simulink model "stage12"  (Simulink 7.7)
settings: Solver=ode45  StartTime=0.0  StopTime=2  RelTol=1e-3
undefined symbols (not defined in the file): Acid, idx_data, iv_data, Lead
libraries: powerlib x23, simulink x4, fl_lib x4, nesl_utility x3, powerlib_extras x2, electricdrivelib x2, elec_lib x2
settings Model: Creator=Vikas  LastModifiedBy=HASANTH

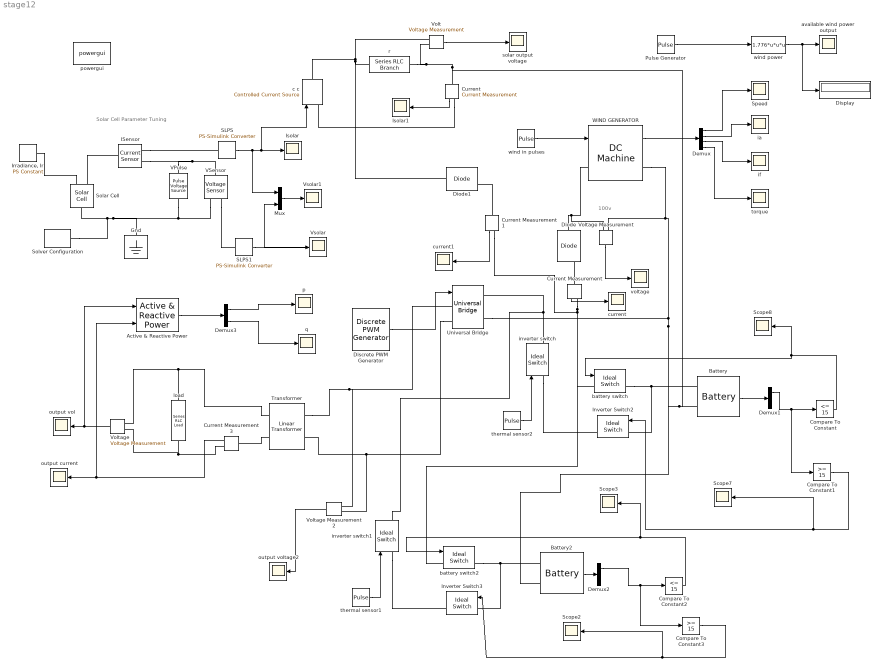
== system stage12 ==
  note: 100v
  note: Solar Cell Parameter Tuning
  Active & Reactive Power : powerlib_extras/Measurements/Active & Reactive Power  SystemSampleTime=-1  f1=50
  Battery : electricdrivelib/Extra Sources/Battery  SystemSampleTime=-1  BatType=Lead-Acid  ShowDetailedParameters=off  NomV=15  NomQ=60  SOC=0  PresetModel=on  MaxQ=62.5  FullV=16.3322  Dis_rate=12  R=0.0025  Normal_OP=18.6167  expZone="[15.2714          0.2]"  Dis_Char=off  current=[6.5 13 32.5]  Units=Time  Batt_Tr=5
  Battery2 : electricdrivelib/Extra Sources/Battery  SystemSampleTime=-1  BatType=Lead-Acid  ShowDetailedParameters=off  NomV=15  NomQ=60  SOC=100  PresetModel=on  MaxQ=62.5  FullV=16.3322  Dis_rate=12  R=0.0025  Normal_OP=18.6167  expZone="[15.2714          0.2]"  Dis_Char=off  current=[6.5 13 32.5]  Units=Time  Batt_Tr=5
  Compare To Constant : simulink/Logic and Bit Operations/Compare To Constant  SystemSampleTime=-1  relop=<=  const=15  LogicOutDataTypeMode=uint8
  Compare To Constant1 : simulink/Logic and Bit Operations/Compare To Constant  SystemSampleTime=-1  relop=>=  const=15  LogicOutDataTypeMode=uint8
  Compare To Constant2 : simulink/Logic and Bit Operations/Compare To Constant  SystemSampleTime=-1  relop=<=  const=15  LogicOutDataTypeMode=uint8
  Compare To Constant3 : simulink/Logic and Bit Operations/Compare To Constant  SystemSampleTime=-1  relop=>=  const=15  LogicOutDataTypeMode=uint8
  Current : powerlib/Measurements/Current Measurement  SystemSampleTime=-1  PhasorSimulation=off  OutputType=Complex  PSBequivalent=0
  Current Measurement : powerlib/Measurements/Current Measurement  SystemSampleTime=-1  PhasorSimulation=off  OutputType=Complex  PSBequivalent=0
  Current Measurement1 : powerlib/Measurements/Current Measurement  SystemSampleTime=-1  PhasorSimulation=off  OutputType=Complex  PSBequivalent=0
  Current Measurement3 : powerlib/Measurements/Current Measurement  SystemSampleTime=-1  PhasorSimulation=off  OutputType=Complex  PSBequivalent=0
  Demux : Demux
  Demux1 : Demux  Outputs=3
  Demux2 : Demux  Outputs=3
  Demux3 : Demux  Outputs=2
  Diode : powerlib/Power Electronics/Diode  SystemSampleTime=-1  Ron=0.001  Lon=0  Vf=0.8  IC=0  UseSnubber=off  Rs=500  Cs=250e-9  Measurements=on
  Diode1 : powerlib/Power Electronics/Diode  SystemSampleTime=-1  Ron=0.001  Lon=0  Vf=0.8  IC=0  UseSnubber=off  Rs=500  Cs=250e-9  Measurements=on
  Discrete PWM Generator : powerlib_extras/Discrete  Control Blocks/Discrete PWM Generator  SystemSampleTime=-1  GeneratorMode="2-arm  bridge (4 pulses)"  Fc=1080  Ts=5e-6  Internal=on  mIndex=0.4  Freq=50  Phase=0
  Display : Display
  Gnd : fl_lib/Electrical/Electrical Elements/Electrical Reference  SystemSampleTime=-1  i_Log=off  LocalVarNames=|i  LocalVarDescs=|i  LocalVarLogging=[]
  ISensor : fl_lib/Electrical/Electrical Sensors/Current Sensor  SystemSampleTime=-1  i1_Log=off  v1_Log=off  LocalVarNames=|i1|v1  LocalVarDescs=|i1|v1  LocalVarLogging=[0 0]
  Inverter Switch2 : powerlib/Power Electronics/Ideal Switch  SystemSampleTime=-1  Ron=0.001  Lon=0  IC=0  Rs=1e5  Cs=inf  Measurements=on
  Inverter Switch3 : powerlib/Power Electronics/Ideal Switch  SystemSampleTime=-1  Ron=0.001  Lon=0  IC=0  Rs=1e5  Cs=inf  Measurements=on
  "Irradiance, Ir" : fl_lib/Physical Signals/Sources/PS Constant  SystemSampleTime=-1  constant=1000  LocalVarLogging=[]
  Isolar : Scope
      settings: TimeRange=1  YMin=2.23577  YMax=2.23577  SaveName=Io
  Isolar1 : Scope
      settings: TimeRange=1  YMin=2.23577  YMax=2.23577  SaveName=Io1
  Mux : Mux  Inputs=2
  Pulse Generator : DiscretePulseGenerator  PulseType=Time based  Amplitude=3.84  Period=10  PulseWidth=50
  SLPS : nesl_utility/PS-Simulink Converter  SystemSampleTime=-1  PhysicalDomain=network_engine_domain  LeftPortType=input  RightPortType=output  SubClassName=ps_output  Unit=A  AffineConversion=off
  SLPS1 : nesl_utility/PS-Simulink Converter  SystemSampleTime=-1  PhysicalDomain=network_engine_domain  LeftPortType=input  RightPortType=output  SubClassName=ps_output  Unit=V  AffineConversion=off
  Scope{2..3,7..8} (4 alike) : Scope
      Scope2 settings: TimeRange=0.1  YMin=0.95  YMax=1.05  SaveName=ScopeData5
      Scope3 settings: TimeRange=0.02  YMin=0.95  YMax=1.05  SaveName=ScopeData10
      Scope7 settings: TimeRange=0.1  YMin=0.95  YMax=1.05  SaveName=ScopeData7
      Scope8 settings: TimeRange=0.02  YMin=0.95  YMax=1.05  SaveName=ScopeData9
  Solar Cell : elec_lib/Sources/Solar Cell  SystemSampleTime=-1  prm=1  Isc=7.34 A  Voc=0.6 V  Is=1e-06 A  Is2=0 A  Iph=7.34 A  Ir0=1000 W/m^2  ec=1.5  N2=2  Rs=0 Ohm  Rp=Inf Ohm  TIPH1=0 1/K  EG=1.11 eV  TXIS1=3  TXIS2=3  TRS1=0  TRP1=0  TFIXED=iv_data(idx_data).temperature C  Tmeas=25 C  LocalVarLogging=[]
  Solver Configuration : nesl_utility/Solver Configuration  SystemSampleTime=-1  PhysicalDomain=network_engine_domain  LeftPortType=input  RightPortType=generic  SubClassName=solver  Accelerate=off  Profile=off  ResidualTolerance=1e-9  MaxNonlinIter=3  MaxModeIter=2  DoFixedCost=off  UseLocalSampling=off  DoDC=off  LinearAlgebra=Sparse  LocalSolverSampleTime=.001  LocalSolverChoice=NE_BACKWARD_EULER_ADVANCER  UseLocalSolver=off
  Speed : Scope
      settings: YMin=5.3  YMax=5.3
  Transformer : powerlib/Elements/Linear Transformer  PhysicalDomain=powersysdomain  SubClassName=unknown  LeftPortType=p1  RightPortType=p1  LConnTagsString=a|b  RConnTagsString=A|B  UNITS=pu  NominalPower=[ 875 50 ]  winding1=[12 0.002 0]  winding2=[240 0.002 0.0]  ThreeWindings=off  winding3=[3.15e+005 0.002 0.08]  RmLm=[500 500]  Measurements=None  DataType=off
  Universal Bridge : powerlib/Power Electronics/Universal Bridge  SystemSampleTime=-1  Arms=2  SnubberResistance=1e5  SnubberCapacitance=inf  Device=MOSFET / Diodes  Ron=1e-3  Lon=0  ForwardVoltages="[  0  0  ]"  ForwardVoltage=0  GTOparameters=[ 10e-6 , 20e-6 ]  IGBTparameters=[ 1e-6 , 2e-6 ]  Measurements=None  Measurements_2=None  converterType=Rectifier
  VPulse : elec_lib/Additional Components/SPICE-Compatible Components/Sources/Pulse Voltage Source  SystemSampleTime=-1  V1=0 V  V2=iv_data(idx_data).v(end) V  TD=0 s  TR=1 s  TF=0 s  PW=Inf s  PER=Inf s  voltage_Log=off  LocalVarNames=|voltage  LocalVarDescs=|Voltage (V)  LocalVarLogging=0
  VSensor : fl_lib/Electrical/Electrical Sensors/Voltage Sensor  SystemSampleTime=-1  i1_Log=off  v1_Log=off  LocalVarNames=|i1|v1  LocalVarDescs=|i1|v1  LocalVarLogging=[0 0]
  Volt : powerlib/Measurements/Voltage Measurement  SystemSampleTime=-1  PhasorSimulation=off  OutputType=Complex  PSBequivalent=0
  Voltage : powerlib/Measurements/Voltage Measurement  SystemSampleTime=-1  PhasorSimulation=off  OutputType=Complex  PSBequivalent=0
  Voltage Measurement : powerlib/Measurements/Voltage Measurement  SystemSampleTime=-1  PhasorSimulation=off  OutputType=Complex  PSBequivalent=0
  Voltage Measurement2 : powerlib/Measurements/Voltage Measurement  SystemSampleTime=-1  PhasorSimulation=off  OutputType=Complex  PSBequivalent=0
  Vsolar : Scope
      settings: TimeRange=1  YMin=0  YMax=0.8  SaveName=Vo
  Vsolar1 : Scope
      settings: TimeRange=1  YMin=0.5  YMax=2.3  SaveName=Vo1
  WIND GENERATOR : powerlib/Machines/DC Machine  SystemSampleTime=-1  PresetModel=No  MechanicalLoad=Speed w  FieldType=Permanent magnet  ShowDetailedParameters=on  RLa="[ 2  0.012]"  RLf="[ 240  120]"  Laf=1.8  MachineConstant=Back-emf constant (V/rpm)  Ke=3  Kt=3.18  J=1  Bm=0  Tf=0  w0=1  Ifinit=1  TsPowergui=0  TsBlock=-1
      settings: AttributesFormatString=\n
  available wind power output : Scope
      settings: TimeRange=0.1  YMin=265.673  YMax=293.639  SaveName=ScopeData13
  battery switch : powerlib/Power Electronics/Ideal Switch  SystemSampleTime=-1  Ron=0.001  Lon=0  IC=0  Rs=1e5  Cs=inf  Measurements=on
  battery switch2 : powerlib/Power Electronics/Ideal Switch  SystemSampleTime=-1  Ron=0.001  Lon=0  IC=0  Rs=1e5  Cs=inf  Measurements=on
  c c : powerlib/Electrical Sources/Controlled Current Source  SystemSampleTime=-1  Initialize=on  Source_Type=DC  Amplitude=1  Phase=0  Frequency=0  Measurements=None
  current : Scope
      settings: TimeRange=0.04  YMin=7.52429  YMax=7.52443  SaveName=ScopeData6
  current1 : Scope
      settings: TimeRange=0.04  YMin=7.21301  YMax=7.21303  SaveName=ScopeData11
  ia : Scope
      settings: YMin=-7.52695  YMax=-7.5266
  if : Scope
      settings: SaveName=ScopeData2
  inverter switch : powerlib/Power Electronics/Ideal Switch  SystemSampleTime=-1  Ron=0.001  Lon=0  IC=0  Rs=1e5  Cs=inf  Measurements=on
  inverter switch1 : powerlib/Power Electronics/Ideal Switch  SystemSampleTime=-1  Ron=0.001  Lon=0  IC=0  Rs=1e5  Cs=inf  Measurements=on
  load : powerlib/Elements/Series RLC Load  PhysicalDomain=powersysdomain  SubClassName=unknown  LeftPortType=p1  RightPortType=p1  LConnTagsString=a  RConnTagsString=__new0  NominalVoltage=230  NominalFrequency=50  ActivePower=500  InductivePower=400  CapacitivePower=100  Setx0=off  InitialVoltage=0  SetiL0=off  InitialCurrent=0  Measurements=None
  output current : Scope
      settings: TimeRange=0.1  YMin=-1.75  YMax=1.75  SaveName=ScopeData15
  output vol : Scope
      settings: YMin=-350  YMax=350  SaveName=ScopeData12
  output voltage2 : Scope
      settings: YMin=-17.5  YMax=17.5  SaveName=ScopeData8
  p : Scope
      settings: TimeRange=1  YMin=-78.75  YMax=-75  SaveName=Vo4
  powergui : powerlib/powergui  Priority=1  SystemSampleTime=-1  SimulationMode=Continuous  SampleTime=50e-6  frequency=60  SPID=off  DisableSnubberDevices=off  DisableRonSwitches=off  DisableVfSwitches=off  SwTol=0  Interpol=off  DisplayEquations=off  FunctionMessages=off  frequencyindice=0  Pbase=100e6  ErrMax=1e-4  Iterations=50  UnitsV=kV  UnitsW=MW  echomessages=off  HookPort=off  EnableUseOfTLC=off  x0status=steady  RestoreLinks=no  ResistiveCurrentMeasurement=off  Frange=[0:2:500]  Ylog=off  Xlog=on  ShowGrid=off  save=off  variable=ZData  structure=ScopeData8  ZoomFFT=off  StartTime=0.0  cycles=1  DisplayStyle=1  fundamental=60  FreqAxis=off  MaxFrequency=1000  frequencyindicesteady=1  RmsSteady=1  display=off  Ts=0  methode=off
  q : Scope
      settings: TimeRange=1  YMin=0  YMax=0.8  SaveName=Vo5
  r : powerlib/Elements/Series RLC Branch  PhysicalDomain=powersysdomain  SubClassName=unknown  LeftPortType=p1  RightPortType=p1  LConnTagsString=__new0  RConnTagsString=__new0  BranchType=R  Resistance=6.75  Inductance=1e-3  SetiL0=off  InitialCurrent=0  Capacitance=1e-6  Setx0=off  InitialVoltage=0  Measurements=None
  solar output voltage : Scope
      settings: YMin=0.853925  YMax=0.85445  SaveName=ScopeData14
  thermal sensor1 : DiscretePulseGenerator  PulseType=Time based  Period=14400  PulseWidth=50
  thermal sensor2 : DiscretePulseGenerator  PulseType=Time based  Period=14400  PulseWidth=50
  torque : Scope
      settings: YMin=-22.6123  YMax=-22.6117  SaveName=ScopeData3
  voltage : Scope
      settings: TimeRange=0.04  YMin=0.8521  YMax=0.85275  SaveName=ScopeData4
  wind in pulses : DiscretePulseGenerator  PulseType=Time based  Amplitude=5.3  Period=10  PulseWidth=50
  "wind power " : Fcn  Expr=1.776*u*u*u
  wires:
  WIND GENERATOR/1 -> Demux/1
  Demux/1 -> Speed/1
  Demux/2 -> ia/1
  Demux/3 -> if/1
  Demux/4 -> torque/1
  Voltage Measurement/1 -> voltage/1
  Battery/1 -> Demux1/1
  Demux1/1 -> Compare To Constant/1, Compare To Constant1/1
  Compare To Constant/1 -> Scope8/1, battery switch/1
  Compare To Constant1/1 -> Inverter Switch2/1, Scope7/1
  Current Measurement/1 -> current/1
  wind in pulses/1 -> WIND GENERATOR/1
  thermal sensor2/1 -> inverter switch/1
  "wind power "/1 -> available wind power output/1, Display/1
  Voltage/1 -> output vol/1, Active & Reactive Power/1
  Voltage Measurement2/1 -> output voltage2/1
  Discrete PWM Generator/1 -> Universal Bridge/1
  Battery2/1 -> Demux2/1
  Demux2/1 -> Compare To Constant2/1, Compare To Constant3/1
  Compare To Constant2/1 -> battery switch2/1, Scope3/1
  Compare To Constant3/1 -> Inverter Switch3/1, Scope2/1
  thermal sensor1/1 -> inverter switch1/1
  SLPS1/1 -> Mux/2, Vsolar/1
  Mux/1 -> Vsolar1/1
  SLPS/1 -> Mux/1, Isolar/1, c c/1
  Current/1 -> Isolar1/1
  Volt/1 -> solar output voltage/1
  Current Measurement3/1 -> output current/1, Active & Reactive Power/2
  Current Measurement1/1 -> current1/1
  Active & Reactive Power/1 -> Demux3/1
  Demux3/1 -> p/1
  Demux3/2 -> q/1
  Pulse Generator/1 -> "wind power "/1
  connections:
  Battery/LConn1 -- battery switch/RConn1 -- Inverter Switch2/LConn1
  Voltage Measurement/LConn1 -- Diode/LConn1 -- WIND GENERATOR/LConn1
  Current Measurement/RConn1 -- battery switch/LConn1 -- battery switch2/LConn1 -- Current Measurement1/RConn1
  inverter switch/LConn1 -- Inverter Switch2/RConn1
  inverter switch1/RConn1 -- Universal Bridge/RConn1 -- inverter switch/RConn1
  load/LConn1 -- Transformer/RConn1 -- Voltage/LConn1
  Universal Bridge/LConn2 -- Transformer/LConn2 -- Voltage Measurement2/LConn2
  Transformer/LConn1 -- Voltage Measurement2/LConn1 -- Universal Bridge/LConn1
  Inverter Switch3/LConn1 -- Battery2/LConn1 -- battery switch2/RConn1
  inverter switch1/LConn1 -- Inverter Switch3/RConn1
  Current Measurement/LConn1 -- Diode/RConn1
  VPulse/RConn1 -- VSensor/RConn2 -- Solver Configuration/RConn1 -- Solar Cell/RConn1 -- Gnd/LConn1
  VPulse/LConn1 -- VSensor/LConn1 -- ISensor/RConn2
  Current/LConn1 -- Volt/LConn2 -- r/LConn1 -- Battery/LConn2 -- Battery2/LConn2 -- Universal Bridge/RConn2 -- Voltage Measurement/LConn2 -- WIND GENERATOR/RConn1
  r/RConn1 -- Volt/LConn1 -- c c/RConn1 -- Diode1/LConn1
  ISensor/RConn1 -- SLPS/LConn1
  Current/RConn1 -- c c/LConn1
  VSensor/RConn1 -- SLPS1/LConn1
  ISensor/LConn1 -- Solar Cell/LConn2
  "Irradiance, Ir"/RConn1 -- Solar Cell/LConn1
  Transformer/RConn2 -- Current Measurement3/LConn1
  Current Measurement3/RConn1 -- load/RConn1 -- Voltage/LConn2
  Current Measurement1/LConn1 -- Diode1/RConn1
